simulink model "eovsa_corr_300mhz"  (R2012b)
(part 10 of 65)

      | %     if length(current_bins) ~= numios,
      | %         error('%d field names specified, but %d binary pts?', numios, length(current_bins));
      | %     end
      | % end
  slice : xbsIndex_r4/Slice  nbits=1  boolean_output=off  mode=Upper Bit Location + Width  bit1=0  base1=MSB of Input  bit0=0  base0=LSB of Input  dbl_ovrd=off  block_type=slice
      settings: block_version=10.1.3
  slice1 : xbsIndex_r4/Slice  nbits=1  boolean_output=off  mode=Upper Bit Location + Width  bit1=-1  base1=MSB of Input  bit0=0  base0=LSB of Input  dbl_ovrd=off  block_type=slice
      settings: block_version=10.1.3
  slice10 : xbsIndex_r4/Slice  nbits=1  boolean_output=on  mode=Lower Bit Location + Width  bit1=-16  base1=MSB of Input  bit0=16  base0=LSB of Input  dbl_ovrd=off  block_type=slice
      settings: block_version=10.1.3
  slice11 : xbsIndex_r4/Slice  nbits=1  boolean_output=on  mode=Lower Bit Location + Width  bit1=0  base1=MSB of Input  bit0=0  base0=LSB of Input  dbl_ovrd=off  block_type=slice
      settings: block_version=10.1.3
  slice12 : xbsIndex_r4/Slice  nbits=4  boolean_output=off  mode=Lower Bit Location + Width  bit1=-16  base1=MSB of Input  bit0=16  base0=LSB of Input  dbl_ovrd=off  block_type=slice
      settings: block_version=10.1.3
  slice13 : xbsIndex_r4/Slice  nbits=16  boolean_output=off  mode=Lower Bit Location + Width  bit1=-16  base1=MSB of Input  bit0=0  base0=LSB of Input  dbl_ovrd=off  block_type=slice
      settings: block_version=10.1.3
  slice14 : xbsIndex_r4/Slice  nbits=1  boolean_output=off  mode=Lower Bit Location + Width  bit1=0  base1=MSB of Input  bit0=0  base0=LSB of Input  dbl_ovrd=off  block_type=slice
      settings: block_version=10.1.3
  slice15 : xbsIndex_r4/Slice  nbits=16  boolean_output=off  mode=Lower Bit Location + Width  bit1=0  base1=MSB of Input  bit0=16  base0=LSB of Input  dbl_ovrd=off  block_type=slice
      settings: block_version=10.1.3
  slice16 : xbsIndex_r4/Slice  nbits=8  boolean_output=off  mode=Lower Bit Location + Width  bit1=0  base1=MSB of Input  bit0=8  base0=LSB of Input  dbl_ovrd=off  block_type=slice
      settings: block_version=10.1.3
  slice17 : xbsIndex_r4/Slice  nbits=4  boolean_output=off  mode=Lower Bit Location + Width  bit1=0  base1=MSB of Input  bit0=4  base0=LSB of Input  dbl_ovrd=off  block_type=slice
      settings: block_version=10.1.3
  slice18 : xbsIndex_r4/Slice  nbits=1  boolean_output=on  mode=Lower Bit Location + Width  bit1=-16  base1=MSB of Input  bit0=8  base0=LSB of Input  dbl_ovrd=off  block_type=slice
      settings: block_version=10.1.3
  slice19 : xbsIndex_r4/Slice  nbits=1  boolean_output=off  mode=Upper Bit Location + Width  bit1=-3  base1=MSB of Input  bit0=0  base0=LSB of Input  dbl_ovrd=off  block_type=slice
      settings: block_version=10.1.3
  slice2 : xbsIndex_r4/Slice  nbits=1  boolean_output=off  mode=Upper Bit Location + Width  bit1=-2  base1=MSB of Input  bit0=0  base0=LSB of Input  dbl_ovrd=off  block_type=slice
      settings: block_version=10.1.3
  slice20 : xbsIndex_r4/Slice  nbits=1  boolean_output=on  mode=Lower Bit Location + Width  bit1=0  base1=MSB of Input  bit0=1  base0=LSB of Input  dbl_ovrd=off  block_type=slice
      settings: block_version=10.1.3
  slice21 : xbsIndex_r4/Slice  nbits=1  boolean_output=on  mode=Lower Bit Location + Width  bit1=-16  base1=MSB of Input  bit0=1  base0=LSB of Input  dbl_ovrd=off  block_type=slice
      settings: block_version=10.1.3
  slice22 : xbsIndex_r4/Slice  nbits=1  boolean_output=on  mode=Lower Bit Location + Width  bit1=-16  base1=MSB of Input  bit0=0  base0=LSB of Input  dbl_ovrd=off  block_type=slice
      settings: block_version=10.1.3
  slice23 : xbsIndex_r4/Slice  nbits=4  boolean_output=off  mode=Lower Bit Location + Width  bit1=-16  base1=MSB of Input  bit0=0  base0=LSB of Input  dbl_ovrd=off  block_type=slice
      settings: block_version=10.1.3
  slice24 : xbsIndex_r4/Slice  nbits=1  boolean_output=on  mode=Upper Bit Location + Width  bit1=0  base1=MSB of Input  bit0=0  base0=LSB of Input  dbl_ovrd=off  block_type=slice
      settings: block_version=10.1.3
  slice3 : xbsIndex_r4/Slice  nbits=1  boolean_output=off  mode=Upper Bit Location + Width  bit1=-8  base1=MSB of Input  bit0=0  base0=LSB of Input  dbl_ovrd=off  block_type=slice
      settings: block_version=10.1.3
  slice4 : xbsIndex_r4/Slice  nbits=1  boolean_output=off  mode=Upper Bit Location + Width  bit1=-9  base1=MSB of Input  bit0=0  base0=LSB of Input  dbl_ovrd=off  block_type=slice
      settings: block_version=10.1.3
  slice5 : xbsIndex_r4/Slice  nbits=1  boolean_output=on  mode=Upper Bit Location + Width  bit1=-10  base1=MSB of Input  bit0=0  base0=LSB of Input  dbl_ovrd=off  block_type=slice
      settings: block_version=10.1.3
  slice6 : xbsIndex_r4/Slice  nbits=1  boolean_output=on  mode=Upper Bit Location + Width  bit1=-11  base1=MSB of Input  bit0=0  base0=LSB of Input  dbl_ovrd=off  block_type=slice
      settings: block_version=10.1.3
  slice7 : xbsIndex_r4/Slice  nbits=1  boolean_output=on  mode=Lower Bit Location + Width  bit1=-16  base1=MSB of Input  bit0=9  base0=LSB of Input  dbl_ovrd=off  block_type=slice
      settings: block_version=10.1.3
  slice8 : xbsIndex_r4/Slice  nbits=12  boolean_output=off  mode=Lower Bit Location + Width  bit1=0  base1=MSB of Input  bit0=16  base0=LSB of Input  dbl_ovrd=off  block_type=slice
      settings: block_version=10.1.3
  slice9 : xbsIndex_r4/Slice  nbits=1  boolean_output=on  mode=Lower Bit Location + Width  bit1=-16  base1=MSB of Input  bit0=0  base0=LSB of Input  dbl_ovrd=off  block_type=slice
      settings: block_version=10.1.3
  snap_select : Subsystem  Tag=xps:sw_reg  AncestorBlock=xps_library/software_register  mask(swreg){mode=one value, io_dir=From Processor, io_delay=0, sample_period=1, names=reg, bitwidths=32, arith_types=0, bin_pts=0, sim_port=on, show_format=off}
      mask prompts: io_dir "I/O direction"; io_delay "I/O delay"; sample_period "Sample period"; names "Name:"; bitwidths "Bitwidth:"; arith_types "Type (ufix=0, fix=1, bool=2):"; bin_pts "Binary pt:"; sim_port "Provide sim input/output?"; show_format "Print format string?"
      mask init:
      | swreg_init(gcb)
      settings: AttributesFormatString=1input
      mask TypeOptions mode: one value | fields of equal size | fields of arbitrary size
      mask Callback mode: swreg_cb(gcb);
      mask TypeOptions io_dir: To Processor | From Processor
      mask Callback io_dir:
      | mask_enables = get_param(gcb, 'MaskEnables');
      | mask_names = get_param(gcb, 'MaskNames');
      | if strcmp(get_param(gcb, 'io_dir'), 'To Processor'),
      |     mask_enables{ismember(mask_names, 'sample_period')} = 'off';
      | else
      |     mask_enables{ismember(mask_names, 'sample_period')} = 'on';
      | end
      | set_param(gcb, 'MaskEnables', mask_enables);
      mask Callback bitwidths:
      | swreg_maskcheck(gcb);
      | % blk = gcb;
      | % mode = get_param(blk, 'mode');
      | % current_widths = eval(get_param(blk, 'bitwidths'));
      | % if (strcmp(mode, 'one value') || strcmp(mode, 'fields of equal size')) && (length(current_widths) > 1),
      | %     error('Only one width may be specified for this mode.');
      | % elseif strcmp(mode, 'fields of arbitrary size')
      | %     current_names = textscan(strtrim(strrep(strrep(get_param(blk, 'names'), ']', ''), '[', '')), '%s');
      | %     current_names = current_names{1};
      | %     numios = length(current_names);
      | %     if length(current_widths) ~= numios,
      | %         error('%d field names specified, but %d widths?', numios, length(current_widths));
      | %     end
      | % end
      | % total_width = 0;
      | % for ctr = 1 : length(current_widths),
      | %     total_width = total_width + current_widths(ctr);
      | % end
      | % if total_width > 32,
      | %     error('Total width must be 32 or less, set to %d.', total_width);
      | % end
      mask Callback arith_types:
      | [numios, ~, ~, ~, current_types] = swreg_maskcheck(gcb);
      | % blk = gcb;
      | % mode = get_param(blk, 'mode');
      | % current_types = eval(get_param(blk, 'arith_types'));
      | % numios = length(current_types);
      | % if (strcmp(mode, 'one value') || strcmp(mode, 'fields of equal size')) && (length(current_types) > 1),
      | %     error('Only one type may be specified for this mode.');
      | % elseif strcmp(mode, 'fields of arbitrary size')
      | %     current_names = textscan(strtrim(strrep(strrep(get_param(blk, 'names'), ']', ''), '[', '')), '%s');
      | %     current_names = current_names{1};
      | %     numios = length(current_names);
      | %     if length(current_types) ~= numios,
      | %         error('%d field names specified, but %d types?', numios, length(current_types));
      | %     end
      | % end
      | problem = 0;
      | for ctr = 1 : numios,
      |     t = current_types(ctr);
      |     if (t < 0) || (t > 2),
      |         problem = t;
      |         ctr = numios + 1;
      |     end
      | end
      | if problem ~= 0,
      |     error('Type cannot be %i, must be 0, 1 or 2.', problem);
      | end
      mask Callback bin_pts:
      | swreg_maskcheck(gcb);
      | % blk = gcb;
      | % mode = get_param(blk, 'mode');
      | % current_bins = eval(get_param(blk, 'bin_pts'));
      | % if (strcmp(mode, 'one value') || strcmp(mode, 'fields of equal size')) && (length(current_bins) > 1),
      | %     error('Only one binary pt may be specified for this mode.');
      | % elseif strcmp(mode, 'fields of arbitrary size')
      | %     current_names = textscan(strtrim(strrep(strrep(get_param(blk, 'names'), ']', ''), '[', '')), '%s');
      | %     current_names = current_names{1};
      | %     numios = length(current_names);
      | %     if length(current_bins) ~= numios,
      | %         error('%d field names specified, but %d binary pts?', numios, length(current_bins));
      | %     end
      | % end
  x_op_select : Subsystem  Tag=xps:sw_reg  AncestorBlock=xps_library/software_register  mask(swreg){mode=one value, io_dir=From Processor, io_delay=0, sample_period=1, names=reg, bitwidths=32, arith_types=0, bin_pts=0, sim_port=on, show_format=off}
      mask prompts: io_dir "I/O direction"; io_delay "I/O delay"; sample_period "Sample period"; names "Name:"; bitwidths "Bitwidth:"; arith_types "Type (ufix=0, fix=1, bool=2):"; bin_pts "Binary pt:"; sim_port "Provide sim input/output?"; show_format "Print format string?"
      mask init:
      | swreg_init(gcb)
      settings: AttributesFormatString=1input
      mask TypeOptions mode: one value | fields of equal size | fields of arbitrary size
      mask Callback mode: swreg_cb(gcb);
      mask TypeOptions io_dir: To Processor | From Processor
      mask Callback io_dir:
      | mask_enables = get_param(gcb, 'MaskEnables');
      | mask_names = get_param(gcb, 'MaskNames');
      | if strcmp(get_param(gcb, 'io_dir'), 'To Processor'),
      |     mask_enables{ismember(mask_names, 'sample_period')} = 'off';
      | else
      |     mask_enables{ismember(mask_names, 'sample_period')} = 'on';
      | end
      | set_param(gcb, 'MaskEnables', mask_enables);
      mask Callback bitwidths:
      | swreg_maskcheck(gcb);
      | % blk = gcb;
      | % mode = get_param(blk, 'mode');
      | % current_widths = eval(get_param(blk, 'bitwidths'));
      | % if (strcmp(mode, 'one value') || strcmp(mode, 'fields of equal size')) && (length(current_widths) > 1),
      | %     error('Only one width may be specified for this mode.');
      | % elseif strcmp(mode, 'fields of arbitrary size')
      | %     current_names = textscan(strtrim(strrep(strrep(get_param(blk, 'names'), ']', ''), '[', '')), '%s');
      | %     current_names = current_names{1};
      | %     numios = length(current_names);
      | %     if length(current_widths) ~= numios,
      | %         error('%d field names specified, but %d widths?', numios, length(current_widths));
      | %     end
      | % end
      | % total_width = 0;
      | % for ctr = 1 : length(current_widths),
      | %     total_width = total_width + current_widths(ctr);
      | % end
      | % if total_width > 32,
      | %     error('Total width must be 32 or less, set to %d.', total_width);
      | % end
      mask Callback arith_types:
      | [numios, ~, ~, ~, current_types] = swreg_maskcheck(gcb);
      | % blk = gcb;
      | % mode = get_param(blk, 'mode');
      | % current_types = eval(get_param(blk, 'arith_types'));
      | % numios = length(current_types);
      | % if (strcmp(mode, 'one value') || strcmp(mode, 'fields of equal size')) && (length(current_types) > 1),
      | %     error('Only one type may be specified for this mode.');
      | % elseif strcmp(mode, 'fields of arbitrary size')
      | %     current_names = textscan(strtrim(strrep(strrep(get_param(blk, 'names'), ']', ''), '[', '')), '%s');
      | %     current_names = current_names{1};
      | %     numios = length(current_names);
      | %     if length(current_types) ~= numios,
      | %         error('%d field names specified, but %d types?', numios, length(current_types));
      | %     end
      | % end
      | problem = 0;
      | for ctr = 1 : numios,
      |     t = current_types(ctr);
      |     if (t < 0) || (t > 2),
      |         problem = t;
      |         ctr = numios + 1;
      |     end
      | end
      | if problem ~= 0,
      |     error('Type cannot be %i, must be 0, 1 or 2.', problem);
      | end
      mask Callback bin_pts:
      | swreg_maskcheck(gcb);
      | % blk = gcb;
      | % mode = get_param(blk, 'mode');
      | % current_bins = eval(get_param(blk, 'bin_pts'));
      | % if (strcmp(mode, 'one value') || strcmp(mode, 'fields of equal size')) && (length(current_bins) > 1),
      | %     error('Only one binary pt may be specified for this mode.');
      | % elseif strcmp(mode, 'fields of arbitrary size')
      | %     current_names = textscan(strtrim(strrep(strrep(get_param(blk, 'names'), ']', ''), '[', '')), '%s');
      | %     current_names = current_names{1};
      | %     numios = length(current_names);
      | %     if length(current_bins) ~= numios,
      | %         error('%d field names specified, but %d binary pts?', numios, length(current_bins));
      | %     end
      | % end
  adc0_atten0 : Outport
  adc0_atten1 : Outport  Port=2
  adc1_atten0 : Outport  Port=3
  adc1_atten1 : Outport  Port=4
  adc0_en0 : Outport  Port=5
  adc0_en1 : Outport  Port=6
  adc1_en0 : Outport  Port=7
  adc1_en1 : Outport  Port=8
  phs_switch0 : Outport  Port=9
  phs_switch1 : Outport  Port=10
  delay00 : Outport  Port=11
  delay01 : Outport  Port=12
  delay10 : Outport  Port=13
  delay11 : Outport  Port=14
  packet_delay : Outport  Port=15
  fft_shift_out : Outport  Port=16
  calibration_bram_address : Outport  Port=17
  calibration_bram_load_data : Outport  Port=18
  calibration_data_x0 : Outport  Port=19
  calibration_data_x1 : Outport  Port=20
  calibration_data_y0 : Outport  Port=21
  calibration_data_y1 : Outport  Port=22
  acc_length : Outport  Port=23
  acc_start_skip : Outport  Port=24
  board_id : Outport  Port=25
  boards_connected : Outport  Port=26
  rst_ten_gbe : Outport  Port=27
  dpp_ip_address : Outport  Port=28
  dpp_port_num : Outport  Port=29
  roach_udp_port : Outport  Port=30
  pps_in : Outport  Port=31
  fpga_pps : Outport  Port=32
  polarization : Outport  Port=33
  adc_protection : Outport  Port=34
  f_x_tvg : Outport  Port=35
  x_eng_tvg : Outport  Port=36
  tvg_rst : Outport  Port=37
  tvg_en : Outport  Port=38
  clr_adc_bad : Outport  Port=39
  clr_status : Outport  Port=40
  input_rst : Outport  Port=41
  input_select : Outport  Port=42
  sw_arm : Outport  Port=43
  x_arm : Outport  Port=44
  reset : Outport  Port=45
  x_acc_length : Outport  Port=46
  x_packet_delay : Outport  Port=47
  x_board_id : Outport  Port=48
  x_rst : Outport  Port=49
  x_polarization : Outport  Port=50
  op_select_x1 : Outport  Port=51
  adc_snap_select : Outport  Port=52
  fft_snap_select : Outport  Port=53
  pol_snap_select : Outport  Port=54
  tx_pkt_snap_select : Outport  Port=55
  rx_hdr_snap_select : Outport  Port=56
  x_in_snap_select : Outport  Port=57
  tag scope: start_mcnt=global, ten_gbe_en=global
  wires:
  acc_len/1(in_reg) -> Delay1/1(d)
  cns_acclen2/1 -> acc_len/1(sim_1)
  Constant22/1 -> arm/1(sim_1)
  arm/1(in_reg) -> Delay6/1(d)
  Constant19/1 -> d0/1(sim_1)
  d0/1(in_reg) -> Delay4/1(d)
  Constant15/1 -> d1/1(sim_1)
  d1/1(in_reg) -> Delay5/1(d)
  phase_switch/1(in_reg) -> Delay2/1(d)
  cns_acclen1/1 -> phase_switch/1(sim_1)
  Constant2/1 -> cal_x0/1(sim_1)
  Constant3/1 -> cal_x1/1(sim_1)
  Constant4/1 -> cal_y0/1(sim_1)
  Constant16/1 -> cal_y1/1(sim_1)
  Constant17/1 -> adc_atten/1(sim_1)
  adc_atten/1(in_reg) -> Delay22/1(d)
  Constant20/1 -> adc_en/1(sim_1)
  adc_en/1(in_reg) -> Delay23/1(d)
  rst/1(in_reg) -> Delay25/1(d)
  err_clear_sim5/1 -> rst/1(sim_1)
  err_clear_sim6/1 -> dpp_ip/1(sim_1)
  err_clear_sim7/1 -> dpp_port/1(sim_1)
  err_clear_sim16/1 -> fx_udp_port/1(sim_1)
  err_clear_sim1/1 -> board_info/1(sim_1)
  Delay2/1(q) -> high16/1, low16/1
  Delay1/1(q) -> low32_17/1, low16_1/1
  Delay5/1(q) -> low16_3/1, high16_3/1
  pkt_fft/1(in_reg) -> Delay3/1(d)
  cns_acclen4/1 -> pkt_fft/1(sim_1)
  Delay3/1(q) -> low_0_7/1, low_0_1/1
  ctrl/1(in_reg) -> Delay76/1(d)
  cns_acclen5/1 -> ctrl/1(sim_1)
  snap_select/1(in_reg) -> Delay50/1(d)
  cns_acclen6/1 -> snap_select/1(sim_1)
  Delay50/1(q) -> low16_6/1, low16_7/1, low16_8/1, low16_13/1, low16_9/1, low16_14/1
  slice5/1 -> edge_detect3/1(in)
  slice6/1 -> edge_detect1/1(in)
  slice7/1 -> edge_detect2/1(in)
  Delay6/1(q) -> slice9/1, slice10/1, slice21/1
  slice9/1 -> edge_detect5/1(in)
  slice10/1 -> edge_detect6/1(in)
  Constant1/1 -> cal_bram/1(sim_1)
  cal_bram/1(in_reg) -> Delay54/1(d)
  cal_x0/1(in_reg) -> Delay7/1(d)
  cal_x1/1(in_reg) -> Delay8/1(d)
  cal_y0/1(in_reg) -> Delay9/1(d)
  cal_y1/1(in_reg) -> Delay10/1(d)
  Delay10/1(q) -> calibration_data_y1/1
  Delay9/1(q) -> calibration_data_y0/1
  Delay8/1(q) -> calibration_data_x1/1
  Delay7/1(q) -> calibration_data_x0/1
  slice8/1 -> calibration_bram_address/1
  slice11/1 -> edge_detect7/1(in)
  high16/1 -> phs_switch0/1
  low16/1 -> phs_switch1/1
  low16_1/1 -> acc_length/1
  low32_17/1 -> acc_start_skip/1
  low_0_7/1 -> packet_delay/1
  low_0_1/1 -> fft_shift_out/1
  low16_2/1 -> delay00/1
  high16_2/1 -> delay01/1
  low16_3/1 -> delay10/1
  high16_3/1 -> delay11/1
  edge_detect5/1(out) -> Delay56/1(d)
  edge_detect6/1(out) -> Delay21/1(d)
  Delay21/1(q) -> reset/1
  Delay56/1(q) -> sw_arm/1
  low16_6/1 -> Delay77/1(d)
  Delay77/1(q) -> adc_snap_select/1
  low16_7/1 -> Delay78/1(d)
  Delay78/1(q) -> fft_snap_select/1
  low16_8/1 -> Delay79/1(d)
  Delay79/1(q) -> pol_snap_select/1
  low16_13/1 -> Delay80/1(d)
  Delay80/1(q) -> tx_pkt_snap_select/1
  low16_9/1 -> Delay81/1(d)
  Delay81/1(q) -> rx_hdr_snap_select/1
  low16_14/1 -> Delay82/1(d)
  Delay82/1(q) -> x_in_snap_select/1
  slice/1 -> Delay74/1(d)
  Delay74/1(q) -> pps_in/1
  slice1/1 -> Delay75/1(d)
  Delay75/1(q) -> fpga_pps/1
  slice2/1 -> Delay83/1(d)
  Delay83/1(q) -> polarization/1
  slice3/1 -> Delay84/1(d)
  Delay84/1(q) -> f_x_tvg/1
  slice4/1 -> Delay85/1(d)
  Delay85/1(q) -> x_eng_tvg/1
  edge_detect3/1(out) -> Delay86/1(d)
  Delay86/1(q) -> tvg_rst/1
  edge_detect1/1(out) -> Delay87/1(d)
  Delay87/1(q) -> tvg_en/1
  edge_detect2/1(out) -> Delay88/1(d)
  Delay88/1(q) -> clr_adc_bad/1
  Delay22/1(q) -> low4/1, low3/1, low1/1, low2/1
  low4/1 -> adc0_atten0/1
  Delay23/1(q) -> low8/1, low7/1, low6/1, low5/1
  low3/1 -> adc0_atten1/1
  low2/1 -> adc1_atten0/1
  low1/1 -> adc1_atten1/1
  low8/1 -> adc0_en0/1
  low7/1 -> adc0_en1/1
  low6/1 -> adc1_en0/1
  low5/1 -> adc1_en1/1
  board_info/1(in_reg) -> Delay24/1(d)
  Delay24/1(q) -> slice12/1, slice13/1
  slice13/1 -> boards_connected/1
  Delay25/1(q) -> Slice6/1
  dpp_ip/1(in_reg) -> Delay26/1(d)
  Delay26/1(q) -> dpp_ip_address/1
  Delay28/1(q) -> dpp_port_num/1
  dpp_port/1(in_reg) -> Delay28/1(d)
  fx_udp_port/1(in_reg) -> Delay112/1(d)
  Delay112/1(q) -> roach_udp_port/1
  Constant24/1 -> ctrl_x/1(sim_1)
  Constant23/1 -> x_op_select/1(sim_1)
  slice14/1 -> Delay120/1(d)
  Delay120/1(q) -> x_polarization/1
  slice15/1 -> Delay121/1(d)
  Delay121/1(q) -> x_acc_length/1
  ctrl_x/1(in_reg) -> Delay11/1(d)
  Delay122/1(q) -> x_packet_delay/1
  slice16/1 -> Delay122/1(d)
  slice17/1 -> Delay123/1(d)
  Delay123/1(q) -> x_board_id/1
  x_op_select/1(in_reg) -> Delay124/1(d)
  Delay124/1(q) -> Delay125/1(d)
  Delay125/1(q) -> op_select_x1/1
  Delay4/1(q) -> low16_2/1, high16_2/1
  slice18/1 -> edge_detect4/1(in)
  edge_detect4/1(out) -> Delay126/1(d)
  Delay126/1(q) -> clr_status/1
  slice19/1 -> Delay127/1(d)
  Delay127/1(q) -> adc_protection/1
  edge_detect7/1(out) -> calibration_bram_load_data/1
  Delay54/1(q) -> slice8/1, slice11/1
  Slice6/1 -> rst_ten_gbe/1
  slice20/1 -> Delay129/1(d)
  Delay129/1(q) -> x_rst/1
  slice12/1 -> board_id/1
  slice21/1 -> edge_detect9/1(in)
  edge_detect9/1(out) -> Delay128/1(d)
  Delay128/1(q) -> x_arm/1
  Constant18/1 -> input_sel/1(sim_1)
  input_sel/1(in_reg) -> Delay133/1(d)
  Delay133/1(q) -> slice24/1, slice23/1
  slice24/1 -> edge_detect10/1(in)
  edge_detect10/1(out) -> Delay132/1(d)
  Delay132/1(q) -> input_rst/1
  Delay130/1(q) -> input_select/1
  slice23/1 -> Delay130/1(d)
  Delay76/1(q) -> slice/1, slice1/1, slice2/1, slice3/1, slice4/1, slice5/1, slice6/1, slice7/1, slice22/1, slice18/1, slice19/1
  Delay134/1(q) -> [ten_gbe_en]
  slice22/1 -> Delay134/1(d)
  Constant21/1 -> mcount_start/1(sim_1)
  mcount_start/1(in_reg) -> Delay135/1(d)
  Delay135/1(q) -> BitBasher/1
  Delay136/1(q) -> [start_mcnt]
  BitBasher/1 -> Delay136/1(d)
  Delay11/1(q) -> slice15/1, slice16/1, slice17/1, slice14/1, slice20/1
